simulink model "frame_3"  (Simulink 7.8)
settings: Solver=FixedStepDiscrete  StartTime=0.0  StopTime=4  RelTol=1e-3
undefined symbols (not defined in the file or in its folder): get
libraries: dspmtrx3 x2, dspbuff3 x1, dspsnks4 x1
settings Model: Creator=svenhoffmann  LastModifiedBy=josef  ExtModeAutoUpdateStatusClock=off
settings OptimizationCC: InitFltsAndDblsToZero=on
settings DebuggingCC: SaveWithParameterizedLinksMsg=none  SignalResolutionControl=TryResolveAllWithWarning  MultiTaskDSMMsg=warning  MultiTaskCondExecSysMsg=none  FcnCallInpInsideContextMsg=Use local settings  StrictBusMsg=None
settings RTWCC: IncludeERTFirstTime=on
settings GRTTargetCC: TargetFcnLib=ansi_tfl_tmw.mat

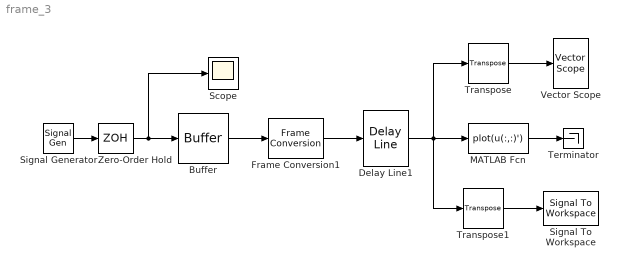
== system frame_3 ==
  Buffer : Buffer
  Delay Line1 : dspbuff3/Delay Line  siz=5  ic=0  directfeed=off  enable_output=off  hold_output=off  TreatMby1Signals=M channels (this choice will be removed - see release notes)
  Frame Conversion1 : FrameConversion  OutFrame=Sample-based
  MATLAB Fcn : MATLABFcn  MATLABFcn=plot(u(:,:)')  OutputSignalType=real  Output1D=off
  Scope : Scope
  Signal Generator : SignalGenerator  WaveForm=sawtooth
  Signal To Workspace : SignalToWorkspace  VariableName=yout  SaveFormat=Array
      settings: CopyFcn=dspblkcopystw(gcbh);
  Terminator : Terminator
  Transpose : dspmtrx3/Transpose  Hermitian=off  overflowFlag=on
  Transpose1 : dspmtrx3/Transpose  Hermitian=off  overflowFlag=on
  Vector Scope : dspsnks4/Vector Scope  ScopeProperties=on  Domain=Time  HorizSpan=1  DisplayProperties=off  AxisGrid=on  Memory=off  FrameNumber=on  AxisLegend=off  AxisZoom=off  OpenScopeAtSimStart=on  OpenScopeImmediately=off  FigPos=get(0,'defaultfigureposition')  AxisProperties=off  XUnits=Hertz  XRange=[0...Fs/2]  InheritXIncr=on  XIncr=1  XLabel=Time  XLimit=Auto  XMin=0  XMax=1  XStart=0  YUnits=dB  YLabel=Amplitude  LineProperties=off  XAxisParamsVer=6.8
      settings: YMin=-0.8463  YMax=-0.1764
  Zero-Order Hold : ZeroOrderHold  SampleTime=1/1000
  wires:
  Signal Generator/1 -> Zero-Order Hold/1
  Zero-Order Hold/1 -> Buffer/1, Scope/1
  Buffer/1 -> Frame Conversion1/1
  Delay Line1/1 -> MATLAB Fcn/1, Transpose/1, Transpose1/1
  MATLAB Fcn/1 -> Terminator/1
  Frame Conversion1/1 -> Delay Line1/1
  Transpose/1 -> Vector Scope/1
  Transpose1/1 -> Signal To Workspace/1
